simulink model "p1_model"  (R2023b)
settings: Solver=VariableStepAuto  StartTime=0.0  StopTime=25  RelTol=1e-3
values from neighbouring files (symbols this model uses):
  A = A_array(l)    [Part2_256_Mostly_Complete.m]    (also in p1_code.m = 1)
  b = b_array(k)    [Part2_256_Mostly_Complete.m]    (also in p1_code.m = 1; project1.m = 10; project1b.m = 10)
  J1 = J1_array(j)    [Part2_256_Mostly_Complete.m]    (also in p1_code.m = 1; project1.m = 100; project1b.m = 100)
  w_0 = w_0_array(i)    [Part2_256_Mostly_Complete.m]    (also in p1_code.m = 1)
settings Model: Creator=natha  LastModifiedBy=natha

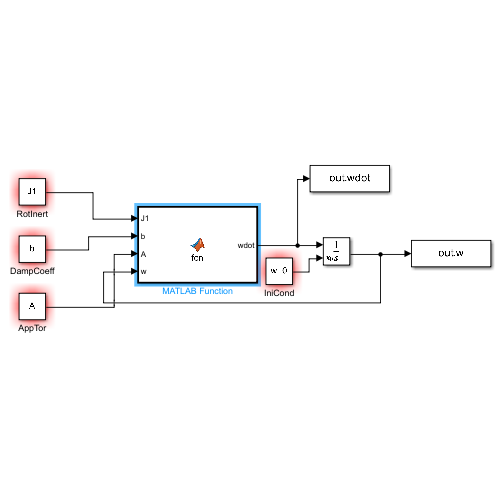
[thumbnail: Simulink's stored preview of the top-level diagram]
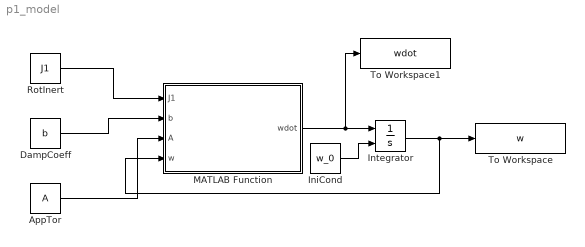
== system p1_model ==
  AppTor : Constant  Value=A
  DampCoeff : Constant  Value=b
  IniCond : Constant  Value=w_0
  Integrator : Integrator  InitialConditionSource=external
  MATLAB Function : MATLAB Function  TreatAsAtomicUnit=on
  RotInert : Constant  Value=J1  SampleTime=-1
  To Workspace : ToWorkspace  VariableName=w  SaveFormat=Timeseries  SampleTime=-1
  To Workspace1 : ToWorkspace  VariableName=wdot  SaveFormat=Timeseries  SampleTime=-1
  wires:
  RotInert/1 -> MATLAB Function/1(J1)
  DampCoeff/1 -> MATLAB Function/2(b)
  AppTor/1 -> MATLAB Function/3(A)
  MATLAB Function/1(wdot) -> To Workspace1/1, Integrator/1
  IniCond/1 -> Integrator/2
  Integrator/1 -> MATLAB Function/4(w), To Workspace/1

== matlab function p1_model/MATLAB Function ==
  data: J1 input; wdot output; b input; A input; w input
function wdot = fcn(J1, b, A, w)

wdot = (1 / J1) * (A - b*w);
